simulink model "wo_buck"  (R2016a)
settings: Solver=VariableStepAuto  StartTime=0.0  StopTime=0.05  RelTol=1e-6
libraries: powerlib x12, simulink x5, powerlib_meascontrol x2
settings Model: Creator=mugino  LastModifiedBy=mugino
settings DebuggingCC: IgnoredZcDiagnostic=none

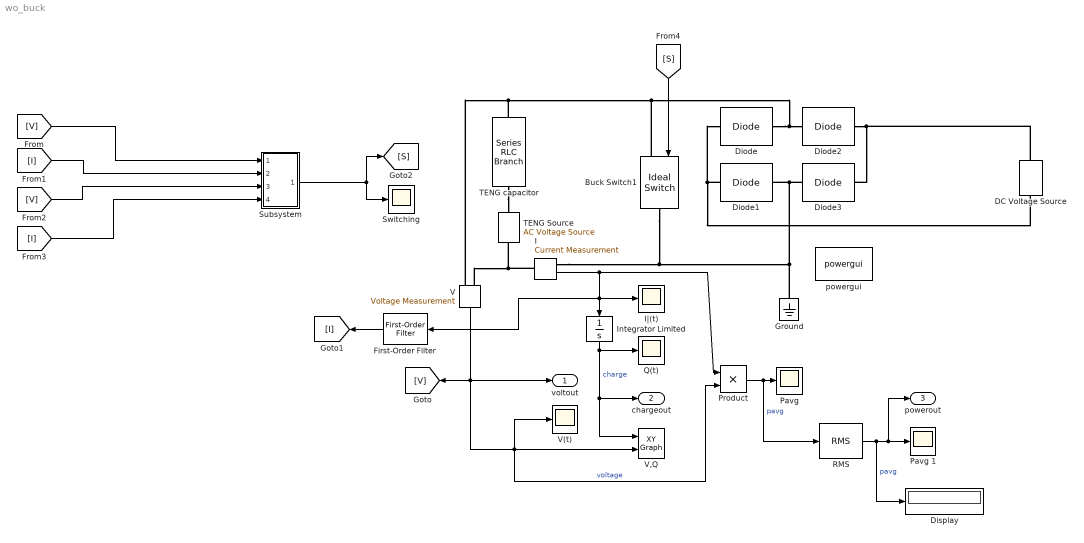
== system wo_buck ==
  Buck Switch1 : powerlib/Power Electronics/Ideal Switch  Ron=0.001  Lon=0  IC=0  Rs=1e6  Cs=inf  Measurements=off
  DC Voltage Source : powerlib/Electrical Sources/DC Voltage Source  Amplitude=200  Measurements=None
  Diode{,1..3} (4 alike) : powerlib/Power Electronics/Diode  Ron=0.001  Lon=1e-3  Vf=0.7  IC=0  UseSnubber=off  Rs=500  Cs=250e-9  Measurements=off
  Display : Display
  First-Order Filter : powerlib_meascontrol/Filters/First-Order Filter  FilterType=Lowpass  Tc=3e-4  Ts=0  Initialize=off  Vac_Init=[0, 0, 60]  Vdc_Init=0  PlotResponse=off  FreqRange="[0,  200,  1]"
  Ground : powerlib/Elements/Ground  LConnTagsString=a
  I : powerlib/Measurements/Current Measurement  PhasorSimulation=off  OutputType=Complex  PSBequivalent=0
  Integrator Limited : Integrator  LimitOutput=on  UpperSaturationLimit=1  LowerSaturationLimit=0  ZeroCross=off
  I|(t) : Scope
  "Pavg " : Scope
  Pavg 1 : Scope
  Product : Product
  Q(t) : Scope
  RMS : powerlib_meascontrol/Measurements/RMS  TrueRMS=on  Freq=50  RMSInit=0  Ts=0
  Subsystem : Subsystem
  "Switching " : Scope
  TENG Source : powerlib/Electrical Sources/AC Voltage Source  Amplitude=310  Phase=0  Frequency=50  SampleTime=0  Measurements=None  BusType=PV  Pref=10e3  Qref=0  Qmin=-inf  Qmax=+inf
  TENG capacitor : powerlib/Elements/Series RLC Branch  LConnTagsString=__new0  RConnTagsString=__new0  BranchType=RC  Resistance=1000  Inductance=1e-7  SetiL0=off  InitialCurrent=0  Capacitance=9e-7  Setx0=off  InitialVoltage=0  Measurements=None
  V : powerlib/Measurements/Voltage Measurement  PhasorSimulation=off  OutputType=Complex  PSBequivalent=0
  V(t) : Scope
  V,Q : simulink/Sinks/XY Graph  xmin=-1e-5  xmax=6e-4  ymin=-300  ymax=300  st=-1
  powergui : powerlib/powergui  Priority=1  SimulationMode=Continuous  SolverType=Tustin/Backward Euler (TBE)  SampleTime=50e-6  frequency=60  SPID=on  DisableSnubberDevices=off  DisableRonSwitches=off  DisableVfSwitches=off  SwTol=0  DisplayEquations=off  Interpol=off  ExternalGateDelay=off  methode=off  Ts=10  FunctionMessages=off  echomessages=off  HookPort=off  EnableUseOfTLC=off  x0status=steady  frequencyindice=0  Pbase=100e6  ErrMax=1e-4  Iterations=50  UnitsV=kV  UnitsW=MW  buscounter=0  RestoreLinks=warning  ResistiveCurrentMeasurement=off  Frange=[0:2:500]  Ylog=off  Xlog=on  ShowGrid=off  save=off  variable=ZData  structure=0  ZoomFFT=off  StartTime=0.0  cycles=1  DisplayStyle=1  fundamental=60  FreqAxis=off  MaxFrequency=1000  frequencyindicesteady=1  RmsSteady=2  display=off
  voltout : Outport
  chargeout : Outport  Port=2
  powerout : Outport  Port=3
  wires:
  Integrator Limited/1 -> chargeout/1, V,Q/1, Q(t)/1  "charge"
  V/1 -> [V], V(t)/1, V,Q/2, Product/2, voltout/1  "voltage"
  I/1 -> Product/1, First-Order Filter/1, I|(t)/1, Integrator Limited/1
  Product/1 -> RMS/1, "Pavg "/1  "pavg"
  RMS/1 -> Display/1, powerout/1, Pavg 1/1  "pavg"
  Subsystem/1(Out1) -> "Switching "/1, [S]
  [V] -> Subsystem/1(In1)
  [I] -> Subsystem/2(In2)
  [V] -> Subsystem/3(In3)
  [I] -> Subsystem/4(In4)
  First-Order Filter/1 -> [I]
  [S] -> Buck Switch1/1
  connections:
  Diode/RConn1 -- Buck Switch1/LConn1 -- TENG capacitor/LConn1 -- V/LConn1 -- Diode2/LConn1
  Diode1/RConn1 -- Diode3/LConn1 -- I/RConn1 -- Buck Switch1/RConn1 -- Ground/LConn1
  TENG Source/LConn1 -- V/LConn2 -- I/LConn1
  Diode1/LConn1 -- DC Voltage Source/LConn1 -- Diode/LConn1
  Diode3/RConn1 -- DC Voltage Source/RConn1 -- Diode2/RConn1
  TENG capacitor/RConn1 -- TENG Source/RConn1

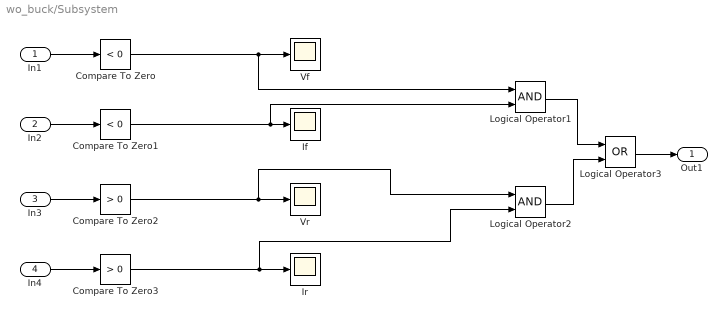
== system wo_buck/Subsystem ==
  In1 : Inport
  In2 : Inport  Port=2
  In3 : Inport  Port=3
  In4 : Inport  Port=4
  Compare To Zero : simulink/Logic and Bit Operations/Compare To Zero  relop=<  OutDataTypeStr=boolean  ZeroCross=off
  Compare To Zero1 : simulink/Logic and Bit Operations/Compare To Zero  relop=<  OutDataTypeStr=boolean  ZeroCross=off
  Compare To Zero2 : simulink/Logic and Bit Operations/Compare To Zero  relop=>  OutDataTypeStr=boolean  ZeroCross=off
  Compare To Zero3 : simulink/Logic and Bit Operations/Compare To Zero  relop=>  OutDataTypeStr=boolean  ZeroCross=off
  If : Scope
  Ir : Scope
  Logical Operator1 : Logic  AllPortsSameDT=off  OutDataTypeStr=boolean
  Logical Operator2 : Logic  AllPortsSameDT=off  OutDataTypeStr=boolean
  Logical Operator3 : Logic  Operator=OR  AllPortsSameDT=off  OutDataTypeStr=boolean
  Vf : Scope
  Vr : Scope
  Out1 : Outport
  wires:
  Logical Operator2/1 -> Logical Operator3/2
  Logical Operator1/1 -> Logical Operator3/1
  In1/1 -> Compare To Zero/1
  Logical Operator3/1 -> Out1/1
  Compare To Zero2/1 -> Logical Operator2/1, Vr/1
  Compare To Zero/1 -> Logical Operator1/1, Vf/1
  In2/1 -> Compare To Zero1/1
  Compare To Zero1/1 -> Logical Operator1/2, If/1
  In3/1 -> Compare To Zero2/1
  In4/1 -> Compare To Zero3/1
  Compare To Zero3/1 -> Logical Operator2/2, Ir/1
